simulink model "buck_test_new"  (R2025a)
settings: Solver=ode14x  StartTime=0.0  StopTime=0.02  FixedStep=1e-6  MaxStep=1e-6  RelTol=1e-3
libraries: spsSeriesRLCBranchLib x3, spsCurrentMeasurementLib x1, spsDCVoltageSourceLib x1, spsDiodeLib x1, spsMosfetLib x1, nesl_utility x1, spsVoltageMeasurementLib x1, sps_lib x1, simulink x1
settings Model: Creator=Edith  LastModifiedBy=HP
settings OptimizationCC: BlockReduction=off  ConditionallyExecuteInputs=off  DefaultParameterBehavior=Inlined
settings DebuggingCC: AlgebraicLoopMsg=error
settings HardwareCC: ProdBitPerPointer=32.0  ProdBitPerSizeT=32.0  ProdBitPerPtrDiffT=32.0  ProdLargestAtomicFloat=None  ProdIntDivRoundTo=Undefined  ProdEndianess=Unspecified  ProdWordSize=32.0  ProdHWDeviceType=ASIC/FPGA->ASIC/FPGA  TargetBitPerPointer=64.0  TargetBitPerSizeT=64.0  TargetBitPerPtrDiffT=64.0  TargetLongLongMode=on  TargetIntDivRoundTo=Zero  TargetEndianess=LittleEndian  TargetWordSize=64.0  TargetHWDeviceType=Custom Processor->MATLAB Host Computer  ProdEqTarget=off

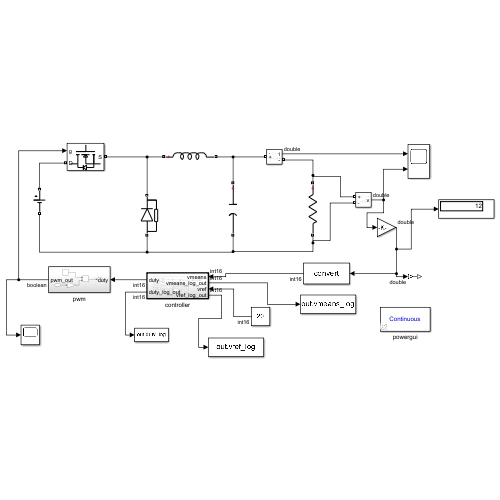
[thumbnail: Simulink's stored preview of the top-level diagram]
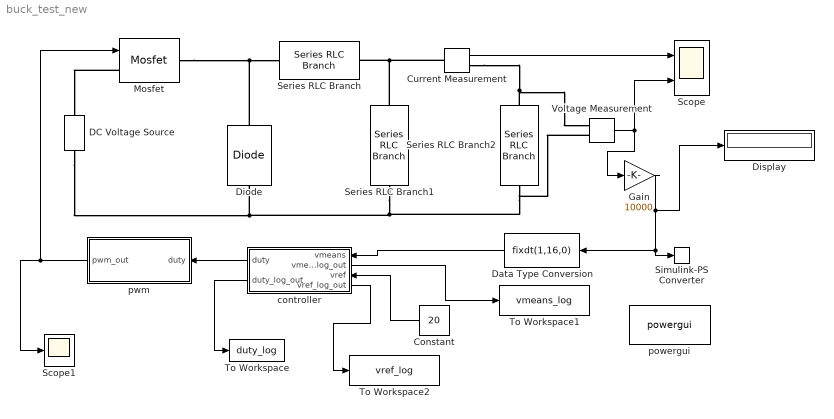
== system buck_test_new ==
  Constant : Constant  Value=20  OutDataTypeStr=fixdt(1,16,0)  SampleTime=-1
  Current Measurement : spsCurrentMeasurementLib/Current Measurement  PhasorSimulation=off  OutputType=Complex  PSBequivalent=0
  DC Voltage Source : spsDCVoltageSourceLib/DC Voltage Source  Amplitude=12  Measurements=None
  Data Type Conversion : DataTypeConversion  OutDataTypeStr=fixdt(1,16,0)  SaturateOnIntegerOverflow=off  RndMeth=Floor
  Diode : spsDiodeLib/Diode  Ron=0.001  Lon=0  Vf=0.8  IC=0  UseSnubber=0  Rs=500  Cs=250e-9  Measurements=off
  Display : Display
  Gain : Gain  Gain=10000
  Mosfet : spsMosfetLib/Mosfet  Ron=0.1  Lon=0  Rd=0.01  Vfd=0  IC=0  Rs=1e5  Cs=inf  Measurements=off
  Scope : Scope  NumInputPorts=2
      settings: ActiveDisplayYMinimum=0.00039995000499949462  ActiveDisplayYMaximum=0.00059995000499949466  YLabel=Output Voltage (V)
  Scope1 : Scope
      settings: ActiveDisplayYMinimum=-0.12499999999999997  ActiveDisplayYMaximum=1.125  YLabel=Pwm signal (0/1)
  Series RLC Branch : spsSeriesRLCBranchLib/Series RLC Branch  LConnTagsString=__new0  RConnTagsString=__new0  BranchType=L  Resistance=1  Inductance=100e-6  SetiL0=off  InitialCurrent=0  Capacitance=1e-6  Setx0=off  InitialVoltage=0  Measurements=None
  Series RLC Branch1 : spsSeriesRLCBranchLib/Series RLC Branch  LConnTagsString=__new0  RConnTagsString=__new0  BranchType=C  Resistance=1  Inductance=1e-3  SetiL0=off  InitialCurrent=0  Capacitance=220e-6  Setx0=off  InitialVoltage=0  Measurements=None
  Series RLC Branch2 : spsSeriesRLCBranchLib/Series RLC Branch  LConnTagsString=__new0  RConnTagsString=__new0  BranchType=R  Resistance=10  Inductance=1e-3  SetiL0=off  InitialCurrent=0  Capacitance=1e-6  Setx0=off  InitialVoltage=0  Measurements=None
  Simulink-PS Converter : nesl_utility/Simulink-PS Converter  PhysicalDomain=network_engine_domain  SubClassName=ps_input  LeftPortType=input  RightPortType=output  PseudoPeriodic=off  Frequencies=[]  NoiseDistribution=none  NoiseParameters=[]  Unit=1  AffineConversion=off  FilteringAndDerivatives=provide  SimscapeFilterOrder=1  InputFilterTimeConstant=0.001  UdotUserProvided=0
  To Workspace : ToWorkspace  VariableName=duty_log  SampleTime=-1
  To Workspace1 : ToWorkspace  VariableName=vmeans_log  SampleTime=-1
  To Workspace2 : ToWorkspace  VariableName=vref_log  SampleTime=-1
  Voltage Measurement : spsVoltageMeasurementLib/Voltage Measurement  PhasorSimulation=off  OutputType=Complex  PSBequivalent=0
  controller : Subsystem  TreatAsAtomicUnit=on  SystemSampleTime=5e-5
      settings: PortSchema="{\"entries\":[{\"content\":{\"sides\":[{\"content\":{\"connectorIds\":[\"In1\",\"Out3\",\"In2\",\"Out4\"]},\"type\":\"ConnectorPlacement.EquallySpacedRectSide\",\"uuid\":\"cb7d65e7-edc4-4cd1-aef4-7ae4c9896b3b\"},{\"content\":{\"connectorIds\":[\"Out1\",\"Out2\"],\"side\":\"RIGHT\"},\"type\":\"ConnectorPlacement.EquallySpacedRectSide\",\"uuid\":\"98099c19-946b-40ba-931b-c3d3ca0c3328\"},{\"content\":{\"side\":\"TOP\"},\"type\":\"ConnectorPlacement.EquallySpacedRectSide\",\"uuid\":\"de5b4eee-403a-406e-b3a4-558d24c53339\"}]},\"type\":\"ConnectorPlacement.EquallySpacedConnector\",\"uuid\":\"6e022ee3-9039-4cf0-abd4-924984288c57\"}],\"packageUris\":[\"http://schema.mathworks.com/mf0/Connector/R2020b\"],\"version\":\"1.0\"}"
  powergui : sps_lib/powergui  Priority=1  SimulationMode=Continuous  SampleTime=50e-6  frequency=60  Iterations=50  frequencyindice=0  Pbase=100e6  ErrMax=1e-4  UnitsV=kV  UnitsW=MW  buscounter=0  FunctionMessages=off  echomessages=off  EnableUseOfTLC=off  CurrentSourceSwitches=off  DisableSnubberDevices=off  DisableRonSwitches=off  DisableVfSwitches=off  DisplayEquations=off  AutomaticDiscreteSolvers=off  SolverType=Tustin/Backward Euler (TBE)  Interpol=off  ExternalGateDelay=off  methode=off  Ts=100  x0status=blocks  SPID=on  SwTol=0  HookPort=off  NonlinearTolerance=1e-4  nMaxIteration=100  ContinueOnMaxIteration=off  RestoreLinks=warning  ResistiveCurrentMeasurement=off  Frange=[0:2:500]  Ylog=off  Xlog=on  ShowGrid=off  save=off  variable=ZData  structure=0  ZoomFFT=off  StartTime=0.0  cycles=1  DisplayStyle=1  fundamental=60  FreqAxis=off  MaxFrequency=1000  frequencyindicesteady=1  RmsSteady=1  display=off
  pwm : Subsystem
  wires:
  Voltage Measurement/1 -> Gain/1, Scope/2
  pwm/1(pwm_out) -> Scope1/1, Mosfet/1
  Constant/1 -> controller/2(vref)
  Data Type Conversion/1 -> controller/1(vmeans)
  controller/1(duty) -> pwm/1(duty)
  controller/4(vref_log_out) -> To Workspace2/1
  controller/3(vmeans_log_out) -> To Workspace1/1
  controller/2(duty_log_out) -> To Workspace/1
  Current Measurement/1 -> Scope/1
  Gain/1 -> Simulink-PS Converter/1, Data Type Conversion/1, Display/1
  connections:
  Diode/RConn1 -- Mosfet/RConn1 -- Series RLC Branch/LConn1
  DC Voltage Source/LConn1 -- Voltage Measurement/LConn2 -- Series RLC Branch2/RConn1 -- Series RLC Branch1/RConn1 -- Diode/LConn1
  Series RLC Branch2/LConn1 -- Voltage Measurement/LConn1 -- Current Measurement/RConn1
  Mosfet/LConn1 -- DC Voltage Source/RConn1
  Series RLC Branch1/LConn1 -- Current Measurement/LConn1 -- Series RLC Branch/RConn1

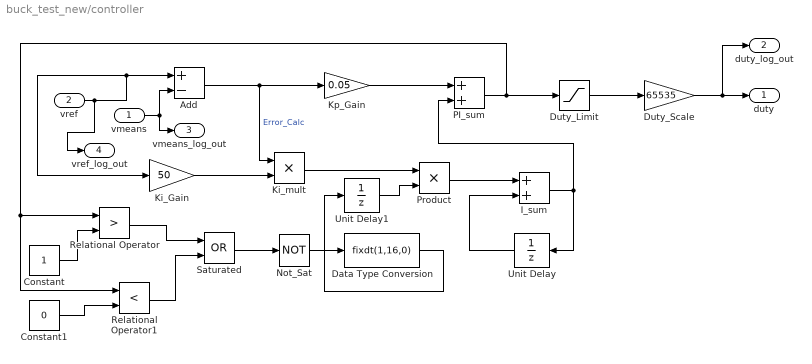
== system buck_test_new/controller ==
  vmeans : Inport  OutDataTypeStr=fixdt(1,16,0)
  vref : Inport  Port=2
  Add : Sum  Inputs=+-  OutDataTypeStr=fixdt(1,16,0)  AccumDataTypeStr=fixdt(1,16,0)
  Constant : Constant  OutDataTypeStr=fixdt(1,16,0)  SampleTime=-1
  Constant1 : Constant  Value=0  OutDataTypeStr=fixdt(1,16,0)  SampleTime=-1
  Data Type Conversion : DataTypeConversion  OutDataTypeStr=fixdt(1,16,0)  SaturateOnIntegerOverflow=off  RndMeth=Floor
  Duty_Limit : Saturate  UpperLimit=1  LowerLimit=0  OutDataTypeStr=fixdt(1,16,0)
  Duty_Scale : Gain  Gain=65535  OutDataTypeStr=fixdt(1,16,0)
  I_sum : Sum  OutDataTypeStr=fixdt(1,16,0)  AccumDataTypeStr=fixdt(1,16,0)
  Ki_Gain : Gain  Gain=50  OutDataTypeStr=fixdt(1,16,0)
  Ki_mult : Product  OutDataTypeStr=fixdt(1,16,0)
  Kp_Gain : Gain  Gain=0.05  OutDataTypeStr=fixdt(1,16,0)
  Not_Sat : Logic  Operator=NOT  AllPortsSameDT=off  OutDataTypeStr=boolean
  PI_sum : Sum  OutDataTypeStr=fixdt(1,16,0)  AccumDataTypeStr=fixdt(1,16,0)
  Product : Product  OutDataTypeStr=fixdt(1,16,0)
  Relational Operator : RelationalOperator  Operator=>  OutDataTypeStr=boolean  RndMeth=Simplest  InputSameDT=off
  Relational Operator1 : RelationalOperator  Operator=<  OutDataTypeStr=boolean  RndMeth=Simplest  InputSameDT=off
  Saturated : Logic  Operator=OR  AllPortsSameDT=off  OutDataTypeStr=boolean
  Unit Delay : UnitDelay  SampleTime=5e-5  HasFrameUpgradeWarning=on
  Unit Delay1 : UnitDelay  SampleTime=-1  HasFrameUpgradeWarning=on
  duty : Outport
  duty_log_out : Outport  Port=2
  vmeans_log_out : Outport  Port=3
  vref_log_out : Outport  Port=4
  wires:
  vref/1 -> vref_log_out/1, Ki_Gain/1, Add/1
  vmeans/1 -> vmeans_log_out/1, Add/2
  Add/1 -> Ki_mult/1, Kp_Gain/1  "Error_Calc"
  Kp_Gain/1 -> PI_sum/1
  Ki_Gain/1 -> Ki_mult/2
  PI_sum/1 -> Relational Operator1/1, Relational Operator/1, Duty_Limit/1
  Not_Sat/1 -> Data Type Conversion/1
  Product/1 -> I_sum/1
  Ki_mult/1 -> Product/1
  Unit Delay/1 -> I_sum/2
  Duty_Limit/1 -> Duty_Scale/1
  Duty_Scale/1 -> duty_log_out/1, duty/1
  I_sum/1 -> Unit Delay/1, PI_sum/2
  Relational Operator1/1 -> Saturated/2
  Relational Operator/1 -> Saturated/1
  Saturated/1 -> Not_Sat/1
  Constant/1 -> Relational Operator/2
  Constant1/1 -> Relational Operator1/2
  Unit Delay1/1 -> Product/2
  Data Type Conversion/1 -> Unit Delay1/1

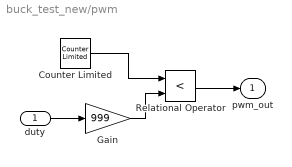
== system buck_test_new/pwm ==
  duty : Inport
  Counter Limited : simulink/Sources/Counter Limited  uplimit=999  tsamp=1e-6
  Gain : Gain  Gain=999  OutDataTypeStr=fixdt(1,16,0)
  Relational Operator : RelationalOperator  Operator=<  OutDataTypeStr=boolean  RndMeth=Simplest  InputSameDT=off
  pwm_out : Outport
  wires:
  Counter Limited/1 -> Relational Operator/1
  Gain/1 -> Relational Operator/2
  duty/1 -> Gain/1
  Relational Operator/1 -> pwm_out/1
